simulink model "Interleaved_Buck_Motor_4"  (R2021a)
settings: Solver=ode23tb  StartTime=0.0  StopTime=0.5  MaxStep=1e-8  RelTol=1e-3
InitFcn:
  | Interleaved_Script
values from neighbouring files (symbols this model uses):
  Cout = 440e-6    (= 0.00044)    [Interleaved_Script.m]
  DCR = 100e-3    (= 0.1)    [Interleaved_Script.m]
  duty_cycle = 0.5    [Interleaved_Script.m]
  EN = 1    [Interleaved_Script.m]
  fs = 20000    [Interleaved_Script.m]
  fsw = 75000    [Interleaved_Script.m]
  ki_v = 1    [Interleaved_Script.m]
  kp_v = 0.0005; S    [Interleaved_Script.m]
  L = 560e-6    (= 0.00056)    [Interleaved_Script.m]
  Tload = 21    [Interleaved_Script.m]
  vref = 120    [Interleaved_Script.m]
libraries: spsCurrentMeasurementLib x7, spsSeriesRLCBranchLib x6, spsVoltageMeasurementLib x6, spsMeanLib x5, spsRMSLib x5, spsDiodeLib x4, spsMosfetLib x4, spsDCVoltageSourceLib x2, spsDCMachineLib x1, spsGroundLib x1, spspowerguiLib x1
settings Model: SimulationMode=rapid-accelerator  Creator=rigas  LastModifiedBy=rigas

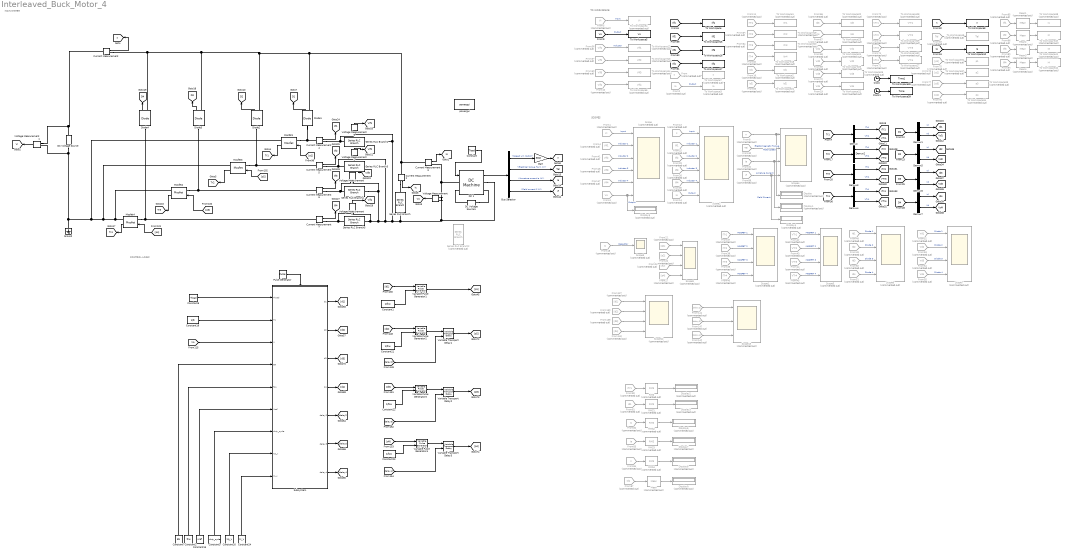
== system Interleaved_Buck_Motor_4 ==
  note: SCOPES
  note: TO WORKSPACE
  note: MAIN SYSTEM
  note: CONTROL LOGIC
  Bus Selector : BusSelector  OutputSignals=Speed wm (rad/s),Electrical torque Te (n m),Armature current ia (A),Field current if (A)
  Clock : Clock
  Clock1 : Clock
  Constant : Constant  Value=Tload
  Constant{1,21..23} (4 alike) : Constant  Value=1/fsw
  Constant15 : Constant  Value=vref
  Constant19 : Constant  Value=1/fs
  Constant2 : Constant  Value=fsw
  Constant20 : Constant  Value=kp_v
  Constant24 : Constant  Value=ki_v
  Constant3 : Constant  Value=duty_cycle
  Constant6 : Constant  Value=Tload
  Constant7 : Constant  Value=EN
  Current Measurement{,2..7} (7 alike) : spsCurrentMeasurementLib/Current Measurement  PhasorSimulation=off  OutputType=Complex  PSBequivalent=0
  DC 1 : spsDCMachineLib/DC Machine  PresetModel=No  MechanicalLoad=Torque TL  FieldType=Wound  ShowDetailedParameters=on  MeasurementBus=off  RLa=[0.83 0.0003]  RLf=[286.64 60]  Laf=2.36  MachineConstant=Torque constant (N.m/A)  Ke=1.8  Kt=1.8  J=0.02  Bm=0.003  Tf=0.58  w0=84  Ifinit=0.5442366731789  TsPowergui=0  TsBlock=-1
  DC Voltage Source : spsDCVoltageSourceLib/DC Voltage Source  Amplitude=240  Measurements=None
  DC Voltage Source1 : spsDCVoltageSourceLib/DC Voltage Source  Amplitude=156  Measurements=None
  Demux{,1..7} (8 alike) : Demux  Outputs=2
  Diode{1..4} (4 alike) : spsDiodeLib/Diode  Ron=0.001  Lon=0  Vf=0.8  IC=0  UseSnubber=0  Rs=500  Cs=250e-9  Measurements=on
  Display{,1..9} (10 alike) : Display  Commented=on
  From : From  Commented=on  GotoTag=Ii  TagVisibility=global
  From1 : From  Commented=on  GotoTag=Vi  TagVisibility=global
  From10 : From  Commented=on  GotoTag=Vlf4  TagVisibility=global
  From11 : From  Commented=on  GotoTag=ITr1  TagVisibility=global
  From13 : From  Commented=on  GotoTag=Ii  TagVisibility=global
  From137 : From  Commented=on  GotoTag=d1
  From138 : From  Commented=on  GotoTag=d2
  From139 : From  Commented=on  GotoTag=d3
  From14 : From  Commented=on  GotoTag=Io  TagVisibility=global
  From140 : From  Commented=on  GotoTag=d4
  From141 : From  Commented=on  GotoTag=delay2
  From142 : From  Commented=on  GotoTag=delay3
  From143 : From  Commented=on  GotoTag=delay4
  From15 : From  Commented=on  GotoTag=Ilf1  TagVisibility=global
  From{16,48,81,87} (4 alike) : From  Commented=on  GotoTag=Id1  TagVisibility=global
  From18 : From  Commented=on  GotoTag=Ic  TagVisibility=global
  From19 : From  Commented=on  GotoTag=Vd4  TagVisibility=global
  From2 : From  Commented=on  GotoTag=Io  TagVisibility=global
  From21 : From  Commented=on  GotoTag=p1
  From22 : From  Commented=on  GotoTag=p2
  From24 : From  Commented=on  GotoTag=p3
  From26 : From  Commented=on  GotoTag=Ilf3  TagVisibility=global
  From27 : From  Commented=on  GotoTag=p4
  From29 : From  Commented=on  GotoTag=Ilf2  TagVisibility=global
  From3 : From  Commented=on  GotoTag=Vo  TagVisibility=global
  From30 : From  Commented=on  GotoTag=Tel  TagVisibility=global
  From31 : From  Commented=on  GotoTag=Ia  TagVisibility=global
  From33 : From  Commented=on  GotoTag=Tel  TagVisibility=global
  From35 : From  Commented=on  GotoTag=Ilf4  TagVisibility=global
  From37 : From  Commented=on  GotoTag=ITr1  TagVisibility=global
  From38 : From  Commented=on  GotoTag=ITr2  TagVisibility=global
  From39 : From  Commented=on  GotoTag=ITr3  TagVisibility=global
  From4 : From  Commented=on  GotoTag=Vlf1  TagVisibility=global
  From40 : From  Commented=on  GotoTag=ITr4  TagVisibility=global
  From41 : From  Commented=on  GotoTag=Vlf2  TagVisibility=global
  From42 : From  Commented=on  GotoTag=VTr1  TagVisibility=global
  From43 : From  Commented=on  GotoTag=VTr2  TagVisibility=global
  From44 : From  Commented=on  GotoTag=VTr3  TagVisibility=global
  From45 : From  Commented=on  GotoTag=VTr4  TagVisibility=global
  From46 : From  Commented=on  GotoTag=Vlf3  TagVisibility=global
  From47 : From  Commented=on  GotoTag=Vlf4  TagVisibility=global
  From49 : From  Commented=on  GotoTag=Id2  TagVisibility=global
  From5 : From  Commented=on  GotoTag=Vi  TagVisibility=global
  From50 : From  Commented=on  GotoTag=Id3  TagVisibility=global
  From51 : From  Commented=on  GotoTag=Id4  TagVisibility=global
  From52 : From  Commented=on  GotoTag=Vd1  TagVisibility=global
  From53 : From  Commented=on  GotoTag=Vd2  TagVisibility=global
  From54 : From  Commented=on  GotoTag=Vd3  TagVisibility=global
  From55 : From  Commented=on  GotoTag=Vd4  TagVisibility=global
  From56 : From  Commented=on  GotoTag=Vlf1  TagVisibility=global
  From57 : From  Commented=on  GotoTag=Vlf2  TagVisibility=global
  From58 : From  Commented=on  GotoTag=Vlf3  TagVisibility=global
  From62 : From  Commented=on  GotoTag=ITr4  TagVisibility=global
  From63 : From  Commented=on  GotoTag=ITr2  TagVisibility=global
  From64 : From  Commented=on  GotoTag=ITr3  TagVisibility=global
  From65 : From  Commented=on  GotoTag=Id2  TagVisibility=global
  From66 : From  Commented=on  GotoTag=Id3  TagVisibility=global
  From67 : From  Commented=on  GotoTag=Id4  TagVisibility=global
  From68 : From  Commented=on  GotoTag=Vd1  TagVisibility=global
  From69 : From  Commented=on  GotoTag=Vd2  TagVisibility=global
  From70 : From  Commented=on  GotoTag=Vd3  TagVisibility=global
  From71 : From  Commented=on  GotoTag=VTr4  TagVisibility=global
  From72 : From  Commented=on  GotoTag=VTr1  TagVisibility=global
  From73 : From  Commented=on  GotoTag=VTr2  TagVisibility=global
  From74 : From  Commented=on  GotoTag=VTr3  TagVisibility=global
  From75 : From  Commented=on  GotoTag=p1
  From76 : From  Commented=on  GotoTag=p2
  From77 : From  Commented=on  GotoTag=p3
  From78 : From  Commented=on  GotoTag=p4
  From8 : From  Commented=on  GotoTag=n  TagVisibility=global
  From80 : From  Commented=on  GotoTag=ITr1  TagVisibility=global
  From82 : From  Commented=on  GotoTag=Ic  TagVisibility=global
  From83 : From  Commented=on  GotoTag=Ia  TagVisibility=global
  From84 : From  Commented=on  GotoTag=Ii  TagVisibility=global
  From85 : From  Commented=on  GotoTag=Ilf1  TagVisibility=global
  From86 : From  Commented=on  GotoTag=Ilf2  TagVisibility=global
  From88 : From  Commented=on  GotoTag=If  TagVisibility=global
  From89 : From  Commented=on  GotoTag=Ilf3  TagVisibility=global
  From90 : From  Commented=on  GotoTag=Ilf4  TagVisibility=global
  Gain : Gain  Gain=30/pi
  Ground : spsGroundLib/Ground  LConnTagsString=a
  Mean{,1..4} (5 alike) : spsMeanLib/Mean  Commented=on  Freq=fsw  Vinit=0  Ts=0
  Mosfet{1..4} (4 alike) : spsMosfetLib/Mosfet  Ron=Ron  Lon=0  Rd=0.01  Vfd=0  IC=0  Rs=1e5  Cs=inf  Measurements=on
  Pulse Generator : DiscretePulseGenerator  PulseType=Time based  Period=1/20000  PulseWidth=50
  RMS{,1..4} (5 alike) : spsRMSLib/RMS  Commented=on  TrueRMS=on  Freq=fsw  RMSInit=0  Ts=0
  Scope : Scope  Commented=on  NumInputPorts=6
  Scope{1,4..7,9,12} (7 alike) : Scope  Commented=on  NumInputPorts=4
  Scope13 : Scope  Commented=on  NumInputPorts=3
  Scope2 : Scope  Commented=on  NumInputPorts=6
  Scope3 : Scope  Commented=on
  Series RLC Branch : spsSeriesRLCBranchLib/Series RLC Branch  LConnTagsString=__new0  RConnTagsString=__new0  BranchType=C  Resistance=1  Inductance=1e-3  SetiL0=off  InitialCurrent=0  Capacitance=Cout  Setx0=off  InitialVoltage=0  Measurements=None
  Series RLC Branch1 : spsSeriesRLCBranchLib/Series RLC Branch  LConnTagsString=__new0  RConnTagsString=__new0  BranchType=RL  Resistance=DCR  Inductance=L  SetiL0=off  InitialCurrent=2  Capacitance=1e-6  Setx0=off  InitialVoltage=0  Measurements=None
  Series RLC Branch2 : spsSeriesRLCBranchLib/Series RLC Branch  Commented=on  LConnTagsString=__new0  RConnTagsString=__new0  BranchType=R  Resistance=20  Inductance=1e-3  SetiL0=off  InitialCurrent=0  Capacitance=Cout  Setx0=off  InitialVoltage=0  Measurements=None
  Series RLC Branch3 : spsSeriesRLCBranchLib/Series RLC Branch  LConnTagsString=__new0  RConnTagsString=__new0  BranchType=RL  Resistance=DCR  Inductance=L  SetiL0=off  InitialCurrent=0  Capacitance=1e-6  Setx0=off  InitialVoltage=0  Measurements=None
  Series RLC Branch4 : spsSeriesRLCBranchLib/Series RLC Branch  LConnTagsString=__new0  RConnTagsString=__new0  BranchType=RL  Resistance=DCR  Inductance=L  SetiL0=off  InitialCurrent=0  Capacitance=1e-6  Setx0=off  InitialVoltage=0  Measurements=None
  Series RLC Branch5 : spsSeriesRLCBranchLib/Series RLC Branch  LConnTagsString=__new0  RConnTagsString=__new0  BranchType=RL  Resistance=DCR  Inductance=L  SetiL0=off  InitialCurrent=0  Capacitance=1e-6  Setx0=off  InitialVoltage=0  Measurements=None
  Subsystem : Subsystem
  To Workspace : ToWorkspace  VariableName=Ilf1  SampleTime=1e-7
  To Workspace1 : ToWorkspace  Commented=on  VariableName=Itr1  SampleTime=-1
  To Workspace10 : ToWorkspace  VariableName=Ia  SampleTime=1e-3
  To Workspace11 : ToWorkspace  Commented=on  VariableName=Vd4  SampleTime=-1
  To Workspace12 : ToWorkspace  Commented=on  VariableName=Vlf1  SampleTime=-1
  To Workspace13 : ToWorkspace  Commented=on  VariableName=Vlf2  SampleTime=-1
  To Workspace14 : ToWorkspace  Commented=on  VariableName=Vlf3  SampleTime=-1
  To Workspace15 : ToWorkspace  VariableName=Ilf2  SampleTime=1e-7
  To Workspace16 : ToWorkspace  VariableName=Ilf3  SampleTime=1e-7
  To Workspace17 : ToWorkspace  VariableName=Ilf4  SampleTime=1e-7
  To Workspace18 : ToWorkspace  Commented=on  VariableName=Itr4  SampleTime=-1
  To Workspace19 : ToWorkspace  Commented=on  VariableName=Itr2  SampleTime=-1
  To Workspace2 : ToWorkspace  Commented=on  VariableName=Id1  SampleTime=-1
  To Workspace20 : ToWorkspace  Commented=on  VariableName=Itr3  SampleTime=-1
  To Workspace21 : ToWorkspace  Commented=on  VariableName=Id2  SampleTime=-1
  To Workspace22 : ToWorkspace  Commented=on  VariableName=Id3  SampleTime=-1
  To Workspace23 : ToWorkspace  Commented=on  VariableName=Id4  SampleTime=-1
  To Workspace24 : ToWorkspace  Commented=on  VariableName=Vd1  SampleTime=-1
  To Workspace25 : ToWorkspace  Commented=on  VariableName=Vd2  SampleTime=-1
  To Workspace26 : ToWorkspace  Commented=on  VariableName=Vd3  SampleTime=-1
  To Workspace27 : ToWorkspace  Commented=on  VariableName=VTr4  SampleTime=-1
  To Workspace28 : ToWorkspace  Commented=on  VariableName=VTr1  SampleTime=-1
  To Workspace29 : ToWorkspace  Commented=on  VariableName=VTr2  SampleTime=-1
  To Workspace3 : ToWorkspace  Commented=on  VariableName=Io  SampleTime=1e-2
  To Workspace30 : ToWorkspace  Commented=on  VariableName=VTr3  SampleTime=-1
  To Workspace31 : ToWorkspace  Commented=on  VariableName=p1  SampleTime=-1
  To Workspace32 : ToWorkspace  Commented=on  VariableName=p2  SampleTime=-1
  To Workspace33 : ToWorkspace  Commented=on  VariableName=p3  SampleTime=-1
  To Workspace34 : ToWorkspace  Commented=on  VariableName=p4  SampleTime=-1
  To Workspace35 : ToWorkspace  VariableName=Time1  SampleTime=1e-3
  To Workspace38 : ToWorkspace  Commented=on  VariableName=I1  SampleTime=1e-6
  To Workspace39 : ToWorkspace  VariableName=Time  SampleTime=1e-7
  To Workspace4 : ToWorkspace  Commented=on  VariableName=Vi  SampleTime=-1
  To Workspace40 : ToWorkspace  Commented=on  VariableName=I2  SampleTime=1e-6
  To Workspace41 : ToWorkspace  Commented=on  VariableName=I3  SampleTime=1e-6
  To Workspace42 : ToWorkspace  Commented=on  VariableName=I4  SampleTime=1e-6
  To Workspace5 : ToWorkspace  VariableName=Vo  SampleTime=1e-3
  To Workspace6 : ToWorkspace  Commented=on  VariableName=Vlf4  SampleTime=-1
  To Workspace7 : ToWorkspace  Commented=on  VariableName=Ii  SampleTime=-1
  To Workspace8 : ToWorkspace  VariableName=n  SampleTime=1e-3
  To Workspace9 : ToWorkspace  Commented=on  VariableName=Tel  SampleTime=-1
  Variable Transport Delay1 : VariableTransportDelay  MaximumDelay=10
  Variable Transport Delay2 : VariableTransportDelay  MaximumDelay=10
  Variable Transport Delay3 : VariableTransportDelay  MaximumDelay=10
  Variable Pulse Generator{1..4} (4 alike) : VariablePulseGenerator  AllowZeroPulseWidth=on  SampleTime=0.1
  Voltage Measurement{,1..5} (6 alike) : spsVoltageMeasurementLib/Voltage Measurement  PhasorSimulation=off  OutputType=Complex  PSBequivalent=0
  powergui : spspowerguiLib/powergui  Priority=1  SimulationMode=Continuous  SampleTime=50e-6  frequency=60  Iterations=50  frequencyindice=0  Pbase=100e6  ErrMax=1e-4  UnitsV=kV  UnitsW=MW  buscounter=0  FunctionMessages=off  echomessages=off  EnableUseOfTLC=off  CurrentSourceSwitches=off  DisableSnubberDevices=off  DisableRonSwitches=off  DisableVfSwitches=off  DisplayEquations=off  AutomaticDiscreteSolvers=off  SolverType=Tustin/Backward Euler (TBE)  Interpol=off  ExternalGateDelay=off  methode=off  Ts=100  x0status=blocks  SPID=on  SwTol=0  HookPort=off  NonlinearTolerance=1e-4  nMaxIteration=100  ContinueOnMaxIteration=off  RestoreLinks=warning  ResistiveCurrentMeasurement=off  Frange=[0:2:500]  Ylog=off  Xlog=on  ShowGrid=off  save=off  variable=ZData  structure=0  ZoomFFT=off  StartTime=0.0  cycles=1  DisplayStyle=1  fundamental=60  FreqAxis=off  MaxFrequency=1000  frequencyindicesteady=1  RmsSteady=1  display=off
  tag scope: D1=global, D2=global, D3=global, D4=global, ITr1=global, ITr2=global, ITr3=global, ITr4=global, Ia=global, Ic=global, Id1=global, Id2=global, Id3=global, Id4=global, If=global, Ii=global, Ilf1=global, Ilf2=global, Ilf3=global, Ilf4=global, Io=global, Tel=global, Tr1=global, Tr2=global, Tr3=global, Tr4=global, VTr1=global, VTr2=global, VTr3=global, VTr4=global, Vd1=global, Vd2=global, Vd3=global, Vd4=global, Vi=global, Vlf1=global, Vlf2=global, Vlf3=global, Vlf4=global, Vo=global, n=global
  wires:
  From88/1 -> Display4/1, Scope4/4  "Field Current"
  [Vo] -> Subsystem/3(V)
  From72/1 -> To Workspace28/1
  From24/1 -> Scope9/3
  From21/1 -> Scope9/1
  From14/1 -> Scope2/6  "Output"
  Demux1/2 -> [Vd1]  "Vd"
  RMS3/1 -> Display7/1
  From5/1 -> To Workspace4/1  "Input"
  Current Measurement2/1 -> [Ic]
  From83/1 -> RMS3/1
  Voltage Measurement4/1 -> [Vlf3]
  RMS1/1 -> Display3/1
  RMS4/1 -> Display8/1
  Demux7/1 -> [Id4]  "Id"
  From77/1 -> To Workspace33/1
  From71/1 -> To Workspace27/1
  From78/1 -> To Workspace34/1
  Variable Transport Delay2/1 -> [p3]
  Variable Transport Delay1/1 -> [p2]
  RMS2/1 -> Display6/1
  Diode4/1 -> [D4]
  From41/1 -> Scope/3  "Inductor 2"
  From10/1 -> To Workspace6/1
  [d4] -> Variable Pulse Generator4/1
  From37/1 -> Scope1/1  "MOSFET 1"
  From63/1 -> To Workspace19/1
  Constant22/1 -> Variable Pulse Generator3/2
  [d1] -> Variable Pulse Generator1/1
  From57/1 -> To Workspace13/1
  From68/1 -> To Workspace24/1
  [Tr3] -> Demux3/1
  From55/1 -> Scope7/4  "Diode 4"
  [D2] -> Demux5/1
  Mosfet1/1 -> [Tr1]
  From11/1 -> To Workspace1/1
  Current Measurement6/1 -> [Ilf3]
  From142/1 -> Scope13/2
  Constant7/1 -> Subsystem/4(EN)
  [Ilf4] -> To Workspace17/1
  Voltage Measurement2/1 -> [Vlf2]
  From62/1 -> To Workspace18/1
  Demux2/2 -> [VTr2]  "VTr1"
  Subsystem/7(delay4) -> [delay4]
  From2/1 -> To Workspace3/1  "Output"
  [Tr2] -> Demux2/1
  Current Measurement5/1 -> [Ilf2]
  From26/1 -> Scope2/4  "Inductor 3"
  From18/1 -> Scope3/1  "Capacitor"
  Diode2/1 -> [D2]
  Demux4/2 -> [VTr4]  "VTr1"
  Voltage Measurement/1 -> [Vo]
  From56/1 -> To Workspace12/1  "Inductor"
  From13/1 -> Scope2/1  "Input"
  From82/1 -> RMS2/1
  Variable Pulse Generator3/1 -> Variable Transport Delay2/1
  From81/1 -> RMS1/1
  Demux6/1 -> [Id3]  "Id"
  [D4] -> Demux7/1
  From47/1 -> Scope/5  "Inductor 4"
  Diode1/1 -> [D1]
  From42/1 -> Scope5/1  "MOSFET 1"
  [D1] -> Demux1/1
  From46/1 -> Scope/4  "Inductor 3"
  Demux7/2 -> [Vd4]  "Vd"
  [Ilf2] -> To Workspace15/1
  Constant1/1 -> Variable Pulse Generator1/2
  From69/1 -> To Workspace25/1
  From35/1 -> Scope2/5  "Inductor 4"
  Constant21/1 -> Variable Pulse Generator2/2
  Demux2/1 -> [ITr2]  "ITr1"
  From33/1 -> To Workspace9/1
  From15/1 -> Scope2/2  "Inductor 1"
  From22/1 -> Scope9/2
  From65/1 -> To Workspace21/1
  Pulse Generator/1 -> Subsystem/Trigger
  From76/1 -> To Workspace32/1
  [n] -> To Workspace8/1
  [Tr4] -> Demux4/1
  From43/1 -> Scope5/2  "MOSFET 2"
  [Ilf1] -> To Workspace/1
  [d2] -> Variable Pulse Generator2/1
  From73/1 -> To Workspace29/1
  Mosfet2/1 -> [Tr3]
  Gain/1 -> [n]
  Subsystem/1(d1) -> [d1]
  [Ilf3] -> To Workspace16/1
  Subsystem/4(d4) -> [d4]
  Subsystem/2(d2) -> [d2]
  From141/1 -> Scope13/1
  Demux5/1 -> [Id2]  "Id"
  From139/1 -> Scope12/3
  From53/1 -> Scope7/2  "Diode 2"
  From137/1 -> Scope12/1
  From16/1 -> To Workspace2/1
  Demux/1 -> [ITr1]  "ITr1"
  Current Measurement/1 -> [Ii]
  Constant20/1 -> Subsystem/8(Kp_v)
  Constant19/1 -> Subsystem/2(Ts)
  [Tr1] -> Demux/1
  Subsystem/5(delay2) -> [delay2]
  DC 1/1 -> Bus Selector/1
  From54/1 -> Scope7/3  "Diode 3"
  From3/1 -> Display5/1, Scope/6  "Output"
  Variable Pulse Generator4/1 -> Variable Transport Delay3/1
  From87/1 -> Mean/1
  Demux3/2 -> [VTr3]  "VTr1"
  From75/1 -> To Workspace31/1
  [p4] -> Mosfet4/1
  From140/1 -> Scope12/4
  Voltage Measurement3/1 -> [Vlf1]
  Variable Transport Delay3/1 -> [p4]
  From8/1 -> Display/1, Scope4/1  "Rotor speed"
  Voltage Measurement5/1 -> [Vlf4]
  From66/1 -> To Workspace22/1
  [delay3] -> Variable Transport Delay2/2
  From40/1 -> Scope1/4  "MOSFET 4"
  From19/1 -> To Workspace11/1
  Demux3/1 -> [ITr3]  "ITr1"
  [p3] -> Mosfet2/1
  From138/1 -> Scope12/2
  Demux1/1 -> [Id1]  "Id"
  From143/1 -> Scope13/3
  Constant24/1 -> Subsystem/9(Ki_v)
  Variable Pulse Generator1/1 -> [p1]
  From27/1 -> Scope9/4
  Voltage Measurement1/1 -> [Vi]
  [Ia] -> To Workspace10/1
  From48/1 -> Scope6/1  "Diode 1"
  From67/1 -> To Workspace23/1
  From50/1 -> Scope6/3  "Diode 3"
  Mosfet3/1 -> [Tr2]
  Current Measurement4/1 -> [Ilf1]
  From/1 -> To Workspace7/1
  [delay4] -> Variable Transport Delay3/2
  From51/1 -> Scope6/4  "Diode 4"
  From29/1 -> Scope2/3  "Inductor 2"
  From38/1 -> Scope1/2  "MOSFET 2"
  Bus Selector/4 -> [If]  "<Field current if (A)>"
  [Vo] -> To Workspace5/1  "Output"
  [p1] -> Mosfet1/1
  RMS/1 -> Display2/1
  Demux6/2 -> [Vd3]  "Vd"
  Bus Selector/1 -> Gain/1  "<Speed wm (rad/s)>"
  From45/1 -> Scope5/4  "MOSFET 4"
  Current Measurement3/1 -> [Io]
  Bus Selector/2 -> [Tel]  "<Electrical torque Te (n m)>"
  From80/1 -> RMS/1
  Variable Pulse Generator2/1 -> Variable Transport Delay1/1
  Constant2/1 -> Subsystem/5(fsw)
  From49/1 -> Scope6/2  "Diode 2"
  From70/1 -> To Workspace26/1
  [D3] -> Demux6/1
  From58/1 -> To Workspace14/1
  Constant23/1 -> Variable Pulse Generator4/2
  From39/1 -> Scope1/3  "MOSFET 3"
  Demux4/1 -> [ITr4]  "ITr1"
  [p2] -> Mosfet3/1
  From44/1 -> Scope5/3  "MOSFET 3"
  Bus Selector/3 -> [Ia]  "<Armature current ia (A)>"
  [delay2] -> Variable Transport Delay1/2
  From74/1 -> To Workspace30/1
  From31/1 -> Display1/1, Scope4/3  "Armature Current"
  From64/1 -> To Workspace20/1
  From52/1 -> Scope7/1  "Diode 1"
  Demux5/2 -> [Vd2]  "Vd"
  From84/1 -> RMS4/1
  From30/1 -> Scope4/2  "Electormagnetic Torque"
  Subsystem/6(delay3) -> [delay3]
  Subsystem/3(d3) -> [d3]
  From4/1 -> Scope/2  "Inductor 1"
  [d3] -> Variable Pulse Generator3/1
  Diode3/1 -> [D3]
  Mean/1 -> Display9/1
  Current Measurement7/1 -> [Ilf4]
  From1/1 -> Scope/1  "Input"
  Mosfet4/1 -> [Tr4]
  Demux/2 -> [VTr1]  "VTr1"
  Clock/1 -> To Workspace35/1
  From85/1 -> Mean1/1
  From89/1 -> Mean3/1
  From86/1 -> Mean2/1
  From90/1 -> Mean4/1
  Mean1/1 -> To Workspace38/1
  Mean3/1 -> To Workspace41/1
  Mean4/1 -> To Workspace42/1
  Mean2/1 -> To Workspace40/1
  Clock1/1 -> To Workspace39/1
  Constant3/1 -> Subsystem/7(duty_cycle)
  Constant15/1 -> Subsystem/6(Vref)
  Constant/1 -> DC 1/1
  Constant6/1 -> Subsystem/1(Tload)
  connections:
  DC Voltage Source/LConn1 -- Ground/LConn1 -- Mosfet1/RConn1 -- Mosfet3/RConn1 -- Mosfet2/RConn1 -- Mosfet4/RConn1 -- Voltage Measurement1/LConn2
  Current Measurement5/RConn1 -- Voltage Measurement2/LConn1 -- Series RLC Branch3/LConn1
  Voltage Measurement/LConn1 -- Current Measurement3/RConn1 -- DC 1/LConn1
  Series RLC Branch4/LConn1 -- Voltage Measurement4/LConn1 -- Current Measurement6/RConn1
  Current Measurement/LConn1 -- Voltage Measurement1/LConn1 -- DC Voltage Source/RConn1
  Series RLC Branch1/LConn1 -- Voltage Measurement3/LConn1 -- Current Measurement4/RConn1
  Current Measurement7/RConn1 -- Voltage Measurement5/LConn1 -- Series RLC Branch5/LConn1
  DC Voltage Source1/RConn1 -- DC 1/LConn2
  Current Measurement2/RConn1 -- Series RLC Branch/LConn1
  DC Voltage Source1/LConn1 -- DC 1/RConn2
  Voltage Measurement3/LConn2 -- Series RLC Branch1/RConn1 -- Series RLC Branch4/RConn1 -- Voltage Measurement4/LConn2 -- Series RLC Branch5/RConn1 -- Voltage Measurement5/LConn2 -- Series RLC Branch3/RConn1 -- Voltage Measurement2/LConn2 -- DC 1/RConn1 -- Voltage Measurement/LConn2 -- Series RLC Branch/RConn1
  Mosfet1/LConn1 -- Diode1/LConn1 -- Current Measurement4/LConn1
  Mosfet3/LConn1 -- Diode2/LConn1 -- Current Measurement5/LConn1
  Mosfet2/LConn1 -- Diode3/LConn1 -- Current Measurement6/LConn1
  Mosfet4/LConn1 -- Diode4/LConn1 -- Current Measurement7/LConn1
  Current Measurement/RConn1 -- Current Measurement3/LConn1 -- Current Measurement2/LConn1 -- Diode1/RConn1 -- Diode2/RConn1 -- Diode3/RConn1 -- Diode4/RConn1

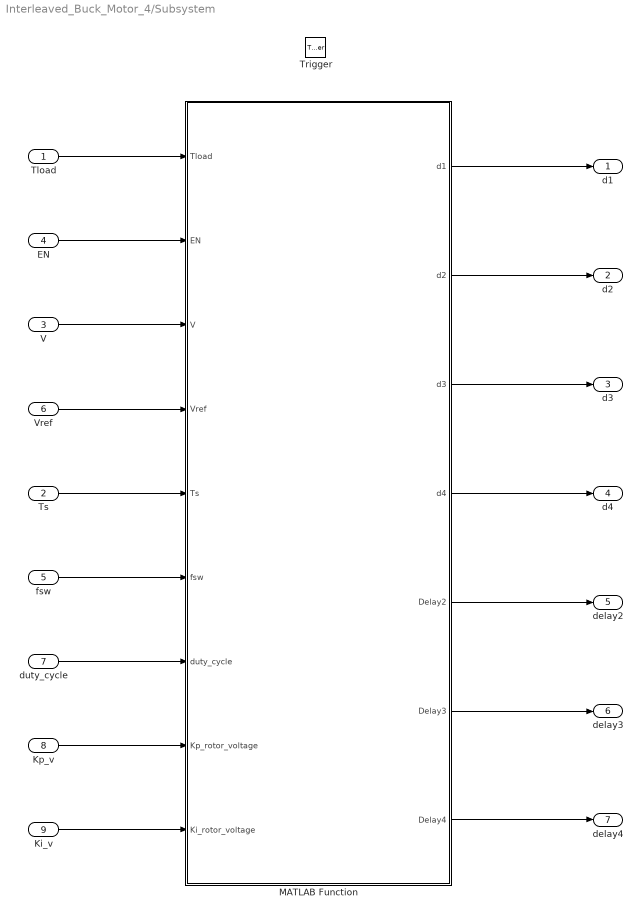
== system Interleaved_Buck_Motor_4/Subsystem ==
  Tload : Inport
  Ts : Inport  Port=2
  V : Inport  Port=3
  EN : Inport  Port=4
  fsw : Inport  Port=5
  Vref : Inport  Port=6
  duty_cycle : Inport  Port=7
  Kp_v : Inport  Port=8
  Ki_v : Inport  Port=9
  Trigger : TriggerPort  VariantControl=(inherit)  PortDimensions=1
  MATLAB Function : MATLAB Function  TreatAsAtomicUnit=on
  d1 : Outport
  d2 : Outport  Port=2
  d3 : Outport  Port=3
  d4 : Outport  Port=4
  delay2 : Outport  Port=5
  delay3 : Outport  Port=6
  delay4 : Outport  Port=7
  wires:
  duty_cycle/1 -> MATLAB Function/7(duty_cycle)
  Ts/1 -> MATLAB Function/5(Ts)
  EN/1 -> MATLAB Function/2(EN)
  V/1 -> MATLAB Function/3(V)
  Vref/1 -> MATLAB Function/4(Vref)
  fsw/1 -> MATLAB Function/6(fsw)
  Tload/1 -> MATLAB Function/1(Tload)
  MATLAB Function/1(d1) -> d1/1
  MATLAB Function/2(d2) -> d2/1
  MATLAB Function/5(Delay2) -> delay2/1
  MATLAB Function/3(d3) -> d3/1
  MATLAB Function/4(d4) -> d4/1
  MATLAB Function/6(Delay3) -> delay3/1
  MATLAB Function/7(Delay4) -> delay4/1
  Kp_v/1 -> MATLAB Function/8(Kp_rotor_voltage)
  Ki_v/1 -> MATLAB Function/9(Ki_rotor_voltage)

== matlab function Interleaved_Buck_Motor_4/Subsystem/MATLAB Function ==
  data: Tload input; d1 output; EN input; V input; Vref input; Ts input; fsw input; duty_cycle input; Kp_rotor_voltage input; Ki_rotor_voltage input; d2 output; d3 output; d4 output; Delay2 output; Delay3 output; Delay4 output
function [d1,d2,d3,d4,Delay2,Delay3,Delay4] = control_unit(Tload,EN,V,Vref,Ts,fsw,duty_cycle,Kp_rotor_voltage,Ki_rotor_voltage)


% ----------- N Calculation ----------%

Ia = 0.7693 * Tload + 0.8394;

% relay 1 %
persistent relay1_state; 
if isempty(relay1_state)
    relay1_state = false;
end
if relay1_state
    if Ia < 3
        relay1_state = false; 
    end
else
    if Ia > 3.5
        relay1_state = true; 
    end
end
if relay1_state
    A = 1;
else
    A = 0;
end

% relay 2 %
persistent relay2_state; 
if isempty(relay2_state)
    relay2_state = false;
end
if relay2_state
    if Ia < 5
        relay2_state = false; 
    end
else
    if Ia > 7
        relay2_state = true; 
    end
end
if relay2_state
    B = 1;
else
    B = 0;
end

% relay 3 %
persistent relay3_state; 
if isempty(relay3_state)
    relay3_state = false;
end
if relay3_state
    if Ia < 7
        relay3_state = false; 
    end
else
    if Ia > 10.5
        relay3_state = true; 
    end
end
if relay3_state
    C = 1;
else
    C = 0;
end

N = 0;
if A == 0
    N = 1;
end
if A == 1 && B == 0
    N = 2;
end
if B == 1 && C == 0
    N = 3;
end
if C == 1
    N = 4;
end

% -------------- Controller Parameters ------&

persistent i_v;
min_output = 0.01;
max_output = 0.99;
kp_v = Kp_rotor_voltage;
ki_v = Ki_rotor_voltage;
error_v = Vref - V;
d1 = 0;
d2 = 0;
d3 = 0;
d4 = 0;
Delay2 = 0;
Delay3 = 0;
Delay4 = 0;

% -------------- Open Loop ---------- %

if EN ==0
    d1 = duty_cycle;
    d2 = duty_cycle;
    d3 = duty_cycle;
    d4 = duty_cycle;
    Delay2 = 0;
    Delay3 = 0;
    Delay4 = 0;
    error_v = 0;
end


% -------------- V PI controller ---------- %

if EN == 1
    if isempty(i_v)
        i_v = 0; 
    end
    error_v = Vref - V;
    p_v = kp_v * error_v;
    new_i_v = i_v + ki_v * error_v * Ts;
    d1_nosat = p_v + new_i_v;
    if d1_nosat > max_output
        d1 = max_output;
        new_i_v = i_v;
    elseif d1_nosat < min_output
        d1 = min_output;
        new_i_v = i_v;
    else
        d1 = d1_nosat;
        i_v = new_i_v;
    end
    i_v = new_i_v;
    d2 = d1;
    d3 = d1;
    d4 = d1;
end


    % -------- Creation of Duty Cycle and Delay for pulses --------%

    % Pulse 1 %
    if d1 > max_output
        d1 = max_output;
    elseif d1 < min_output
        d1 = min_output;
    end

    % Pulse 2 %
    if A > 0 
        if d2 > max_output
            d2 = max_output;
        elseif d2 < min_output
            d2 = min_output;
        end
    else
        d2 = 0;
    end
    Delay2 = (1/N)*(1/fsw);

    % Pulse 3 %
    if B > 0
        if d3 > max_output
            d3 = max_output;
        elseif d3 < min_output
            d3 = min_output;
        end
    else
        d3 = 0;
    end
    Delay3 = (2/N)*(1/fsw);

    % Pulse 4 %
    if C > 0
        if d4 > max_output
            d4 = max_output;
        elseif d4 < min_output
            d4 = min_output;
        end
    else
        d4 = 0;
    end
    Delay4 = (3/N)*(1/fsw);
end
